simulink model "control_stateretroazione"  (R2015a)
settings: Solver=ode45  StartTime=0.0  StopTime=50  RelTol=1e-3
PreLoadFcn:
  | parameters
values from neighbouring files (symbols this model uses):
  Ass = [-R/L, 0, -gamma/M1; 0,0,1; gamma/(2*L), -Kh/M1,-Ch/M1]    [controller.m]
  Bss = [1;0;0]    [controller.m]
  Css = [0,1/M1,0]    [controller.m]
  Kx = place(Ass,Bss,[-100, -70,-50])    [controller.m]
  Lx = place(Ass',Css',[-200,-150,-100])'    [controller.m]
undefined symbols (not defined in the file or in its folder): Ch, D, Ke, Kh, L, M1, R
settings Model: Creator=dell  LastModifiedBy=dell

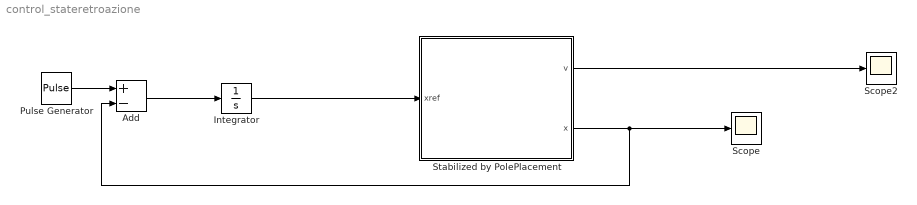
== system control_stateretroazione ==
  Add : Sum  Inputs=+-
  Integrator : Integrator
  Pulse Generator : DiscretePulseGenerator  PulseType=Time based  Period=10  PulseWidth=50
  Scope : Scope
      settings: TimeRange=8  YMin=-1  YMax=1
  Scope2 : Scope
      settings: TimeRange=20  YMin=1.5e-06  YMax=5.75e-06  SaveName=ScopeData3
  Stabilized by PolePlacement : Subsystem
  wires:
  Pulse Generator/1 -> Add/1
  Add/1 -> Integrator/1
  Integrator/1 -> Stabilized by PolePlacement/1(xref)
  Stabilized by PolePlacement/1(v) -> Scope2/1
  Stabilized by PolePlacement/2(x) -> Add/2, Scope/1

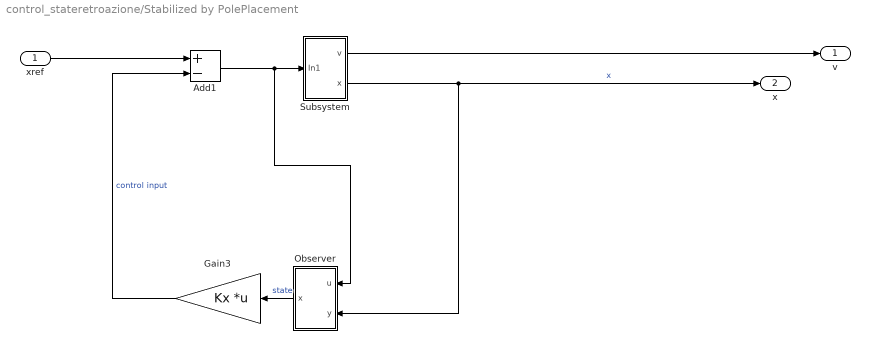
== system control_stateretroazione/Stabilized by PolePlacement ==
  xref : Inport
  Add1 : Sum  Inputs=+-
  Gain3 : Gain  Gain=Kx  Multiplication=Matrix(K*u)
  "Observer " : Subsystem
  Subsystem : Subsystem
  v : Outport
  x : Outport  Port=2
  wires:
  "Observer "/1(x) -> Gain3/1  "state"
  xref/1 -> Add1/1
  Subsystem/1(v) -> v/1
  Add1/1 -> Subsystem/1(In1), "Observer "/1(u)
  Subsystem/2(x) -> x/1, "Observer "/2(y)  "x"
  Gain3/1 -> Add1/2  "control input"

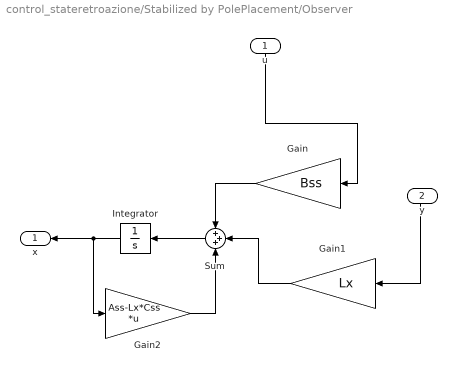
== system control_stateretroazione/Stabilized by PolePlacement/Observer  ==
  u : Inport
  y : Inport  Port=2
  Gain : Gain  Gain=Bss
  Gain1 : Gain  Gain=Lx
  Gain2 : Gain  Gain=Ass-Lx*Css  Multiplication=Matrix(K*u)
  Integrator : Integrator
  Sum : Sum  Inputs=+++
  x : Outport
  wires:
  Sum/1 -> Integrator/1
  y/1 -> Gain1/1
  u/1 -> Gain/1
  Gain2/1 -> Sum/3
  Integrator/1 -> x/1, Gain2/1
  Gain/1 -> Sum/1
  Gain1/1 -> Sum/2

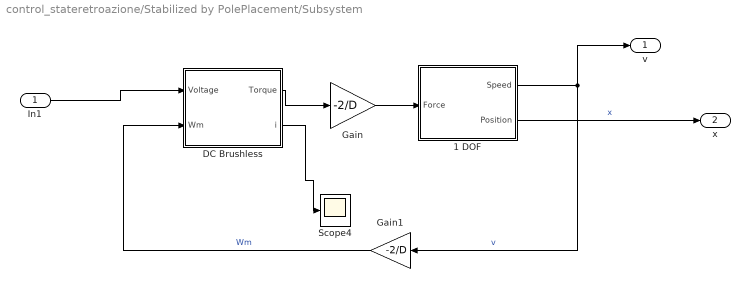
== system control_stateretroazione/Stabilized by PolePlacement/Subsystem ==
  In1 : Inport
  "1 DOF " : Subsystem
  DC Brushless : Subsystem
  Gain : Gain  Gain=-2/D
  Gain1 : Gain  Gain=-2/D
  Scope4 : Scope
      settings: TimeRange=20  YMin=1.5e-06  YMax=5.75e-06  SaveName=ScopeData6
  v : Outport
  x : Outport  Port=2
  wires:
  In1/1 -> DC Brushless/1("Voltage ")
  DC Brushless/1("Torque ") -> Gain/1
  "1 DOF "/1("Speed ") -> v/1, Gain1/1  "v"
  DC Brushless/2("i ") -> Scope4/1
  "1 DOF "/2("Position ") -> x/1  "x"
  Gain1/1 -> DC Brushless/2(Wm)  "Wm"
  Gain/1 -> "1 DOF "/1(Force)

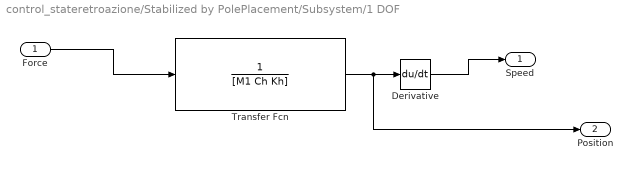
== system control_stateretroazione/Stabilized by PolePlacement/Subsystem/1 DOF  ==
  Force : Inport
  Derivative : Derivative
  Transfer Fcn : TransferFcn  Denominator=[M1 Ch Kh]
  "Speed " : Outport
  "Position " : Outport  Port=2
  wires:
  Force/1 -> Transfer Fcn/1
  Transfer Fcn/1 -> "Position "/1, Derivative/1
  Derivative/1 -> "Speed "/1

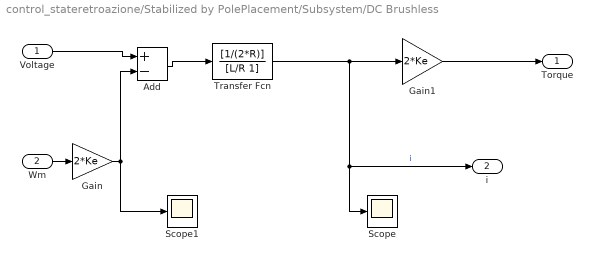
== system control_stateretroazione/Stabilized by PolePlacement/Subsystem/DC Brushless ==
  "Voltage " : Inport
  Wm : Inport  Port=2
  Add : Sum  Inputs=+-
  Gain : Gain  Gain=2*Ke
  Gain1 : Gain  Gain=2*Ke
  Scope : Scope
      settings: YMin=-0.075  YMax=0.125  SaveName=ScopeData2
  Scope1 : Scope
      settings: YMin=-0.35  YMax=0.35  SaveName=ScopeData4
  Transfer Fcn : TransferFcn  Numerator=[1/(2*R)]  Denominator=[L/R 1]
  "Torque " : Outport
  "i " : Outport  Port=2
  wires:
  Gain1/1 -> "Torque "/1
  Transfer Fcn/1 -> "i "/1, Scope/1, Gain1/1  "i"
  Add/1 -> Transfer Fcn/1
  "Voltage "/1 -> Add/1
  Wm/1 -> Gain/1
  Gain/1 -> Scope1/1, Add/2
